simulink model "MRAC2016"  (R2016b)
settings: Solver=ode4  StartTime=0.0  StopTime=10  FixedStep=0.01  MaxStep=1e-3  RelTol=1e-3  AbsTol=1e-4
values from neighbouring files (symbols this model uses):
  A = [-3.1074 0.9744;0.4501 -4.1003]    [MRAC_params.m]
  A_hat_0 = [-5,0.2;0.1,-1]    [MRAC_params.m]
  Am = [-3.3808 1.2954;0.4444 -3.0501]    [MRAC_params.m]
  B = [B1,B2]    [MRAC_params.m]
  beta_1 = 100    [MRAC_params.m]
  Bm = [Bm1,Bm2]    [MRAC_params.m]
  d = [0.21;0.44]    [MRAC_params.m]
  d_hat_0 = [0.08;0.12]    [MRAC_params.m]
  dm = [0.1;0.3]    [MRAC_params.m]
  flag = 1    [MRAC_params.m]
  Gamma_A = 0.01*eye(2)    [MRAC_params.m]
  gamma_A = 0.0001    [MRAC_params.m]
  gamma_d = 1    [MRAC_params.m]
  P = are(Am,zeros(2,2),Q)    [MRAC_params.m]
  x_0 = [0.5;0.2]    [MRAC_params.m]
  xm_0 = [0;0]    [MRAC_params.m]
undefined symbols (not defined in the file or in its folder): sigbuilder_block
settings Model: Creator=RUZHOU  LastModifiedBy=Administrator
settings OptimizationCC: LifeSpan=inf
settings DebuggingCC: SFExecutionAtInitializationDiag=none
settings SFSimCC: SimUseLocalCustomCode=on
settings RTWCC: RTWUseLocalCustomCode=on

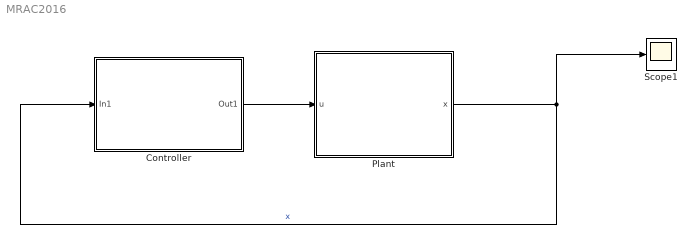
== system MRAC2016 ==
  Controller : Subsystem
  Plant : Subsystem
  Scope1 : Scope
  wires:
  Plant/1(x) -> Controller/1(In1), Scope1/1  "x"
  Controller/1(Out1) -> Plant/1(u)

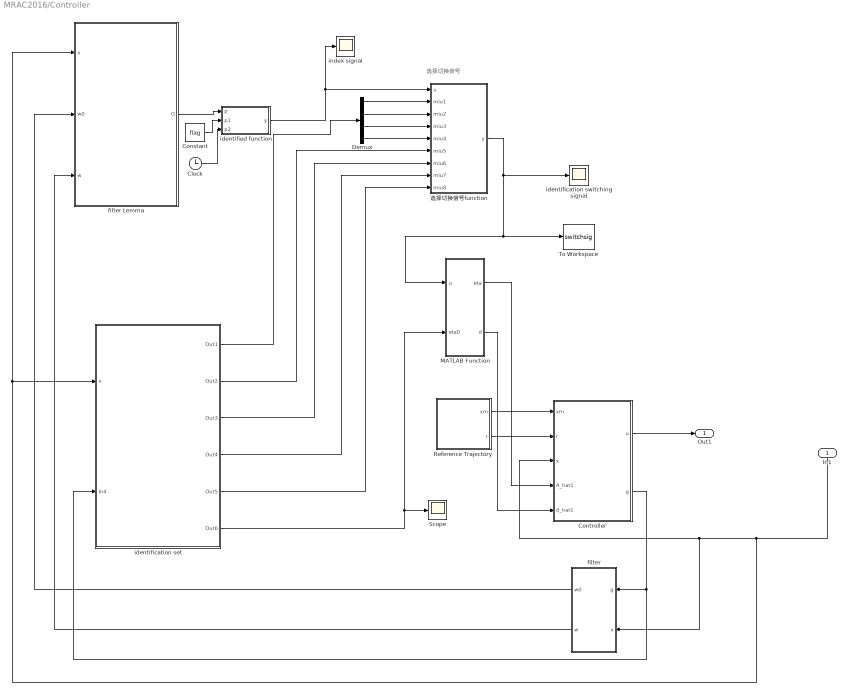
== system MRAC2016/Controller ==
  note: 选择切换信号
  In1 : Inport
  Clock : Clock
  Constant : Constant  Value=flag
  Controller : Subsystem
  Demux : Demux
  MATLAB Function : MATLAB Function  TreatAsAtomicUnit=on
  Reference Trajectory : Subsystem
  Scope : Scope
  To Workspace : ToWorkspace  VariableName=switchsig  SampleTime=-1
      settings: Save2DSignal=2-D array (concatenate along first dimension)
  filter : Subsystem
  filter Lemma : Subsystem
  identification set : Subsystem
  identification switching signal : Scope
  identified function : MATLAB Function  TreatAsAtomicUnit=on
  index signal : Scope
  选择切换信号function : MATLAB Function  TreatAsAtomicUnit=on
  Out1 : Outport
  wires:
  Demux/2 -> 选择切换信号function/3(miu2)
  Demux/3 -> 选择切换信号function/4(miu3)
  Reference Trajectory/2(r) -> Controller/2(r)
  Reference Trajectory/1(xm) -> Controller/1(xm)
  Controller/2(g) -> filter/1("g "), identification set/2(In4)
  Demux/1 -> 选择切换信号function/2(miu1)
  选择切换信号function/1(y) -> identification switching signal/1, To Workspace/1, MATLAB Function/1(u)
  identification set/5(Out5) -> 选择切换信号function/9(miu8)
  Constant/1 -> identified function/2(p1)
  Demux/4 -> 选择切换信号function/5(miu4)
  MATLAB Function/2(d) -> Controller/5(d_hat1)
  MATLAB Function/1(eta) -> Controller/4(A_hat1)
  identification set/1(Out1) -> Demux/1
  filter/1(w0) -> filter Lemma/2(w0)
  identified function/1(y) -> index signal/1, 选择切换信号function/1(u)
  filter/2(w) -> filter Lemma/3(w)
  filter Lemma/1(G) -> identified function/1(p)
  Clock/1 -> identified function/3(p2)
  identification set/4(Out4) -> 选择切换信号function/8(miu7)
  Controller/1(u) -> Out1/1
  identification set/6(Out6) -> Scope/1, MATLAB Function/2(eta0)
  identification set/2(Out2) -> 选择切换信号function/6(miu5)
  identification set/3(Out3) -> 选择切换信号function/7(miu6)
  In1/1 -> identification set/1(x), filter Lemma/1(x), Controller/3(x), filter/2(x)

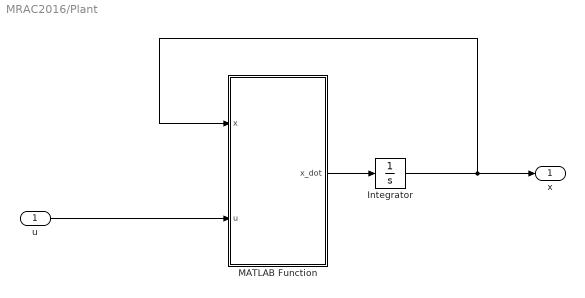
== system MRAC2016/Plant ==
  u : Inport
  Integrator : Integrator  InitialCondition=x_0  LimitOutput=on  UpperSaturationLimit=1000  LowerSaturationLimit=-1000
  MATLAB Function : MATLAB Function  TreatAsAtomicUnit=on
  x : Outport
  wires:
  MATLAB Function/1(x_dot) -> Integrator/1
  Integrator/1 -> MATLAB Function/1(x), x/1
  u/1 -> MATLAB Function/2(u)

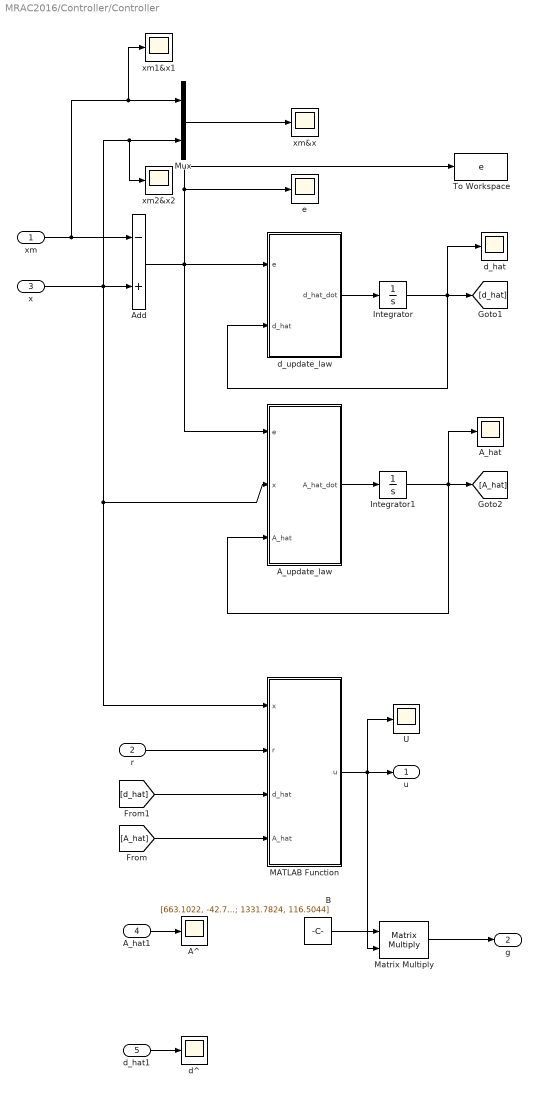
== system MRAC2016/Controller/Controller ==
  xm : Inport
  r : Inport  Port=2
  x : Inport  Port=3
  A_hat1 : Inport  Port=4
  d_hat1 : Inport  Port=5
  A^ : Scope
  A_hat : Scope
  A_update_law : MATLAB Function  TreatAsAtomicUnit=on
  Add : Sum  Inputs=-+
  B : Constant  Value=[663.1022, -42.7; 1331.7824, 116.5044]  VectorParams1D=off
  Integrator : Integrator  InitialCondition=d_hat_0
  Integrator1 : Integrator  InitialCondition=A_hat_0
  MATLAB Function : MATLAB Function  TreatAsAtomicUnit=on
  Matrix Multiply : Product  Multiplication=Matrix(*)
  Mux : Mux  Inputs=2
  To Workspace : ToWorkspace  VariableName=e  SaveFormat=Timeseries  SampleTime=-1
  U : Scope
  d^ : Scope
  d_hat : Scope
  d_update_law : MATLAB Function  TreatAsAtomicUnit=on
  e : Scope
  xm&x : Scope
  xm1&x1 : Scope
  xm2&x2 : Scope
  u : Outport
  g : Outport  Port=2
  wires:
  x/1 -> xm2&x2/1, Mux/2, MATLAB Function/1(x), A_update_law/2(x), Add/2
  xm/1 -> xm1&x1/1, Mux/1, Add/1
  Add/1 -> To Workspace/1, e/1, A_update_law/1(e), d_update_law/1(e)
  d_update_law/1(d_hat_dot) -> Integrator/1
  Integrator/1 -> d_hat/1, d_update_law/2(d_hat), [d_hat]
  A_update_law/1(A_hat_dot) -> Integrator1/1
  Integrator1/1 -> A_update_law/3(A_hat), [A_hat], A_hat/1
  r/1 -> MATLAB Function/2(r)
  [d_hat] -> MATLAB Function/3(d_hat)
  MATLAB Function/1(u) -> Matrix Multiply/2, U/1, u/1
  Mux/1 -> xm&x/1
  B/1 -> Matrix Multiply/1
  Matrix Multiply/1 -> g/1
  A_hat1/1 -> A^/1
  d_hat1/1 -> d^/1
  [A_hat] -> MATLAB Function/4(A_hat)

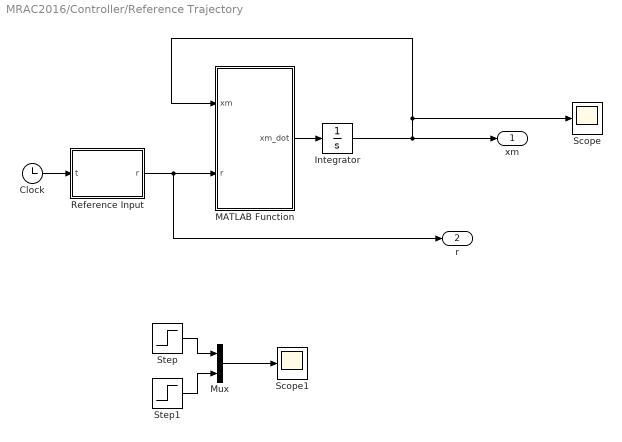
== system MRAC2016/Controller/Reference Trajectory ==
  Clock : Clock
  Integrator : Integrator  InitialCondition=xm_0
  MATLAB Function : MATLAB Function  TreatAsAtomicUnit=on
  Mux : Mux  Inputs=2
  Reference Input : MATLAB Function  TreatAsAtomicUnit=on
  Scope : Scope
  Scope1 : Scope
  Step : Step  SampleTime=0
  Step1 : Step  SampleTime=0
  xm : Outport
  r : Outport  Port=2
  wires:
  MATLAB Function/1(xm_dot) -> Integrator/1
  Clock/1 -> Reference Input/1(t)
  Integrator/1 -> Scope/1, MATLAB Function/1(xm), xm/1
  Reference Input/1(r) -> r/1, MATLAB Function/2(r)
  Step/1 -> Mux/1
  Step1/1 -> Mux/2
  Mux/1 -> Scope1/1

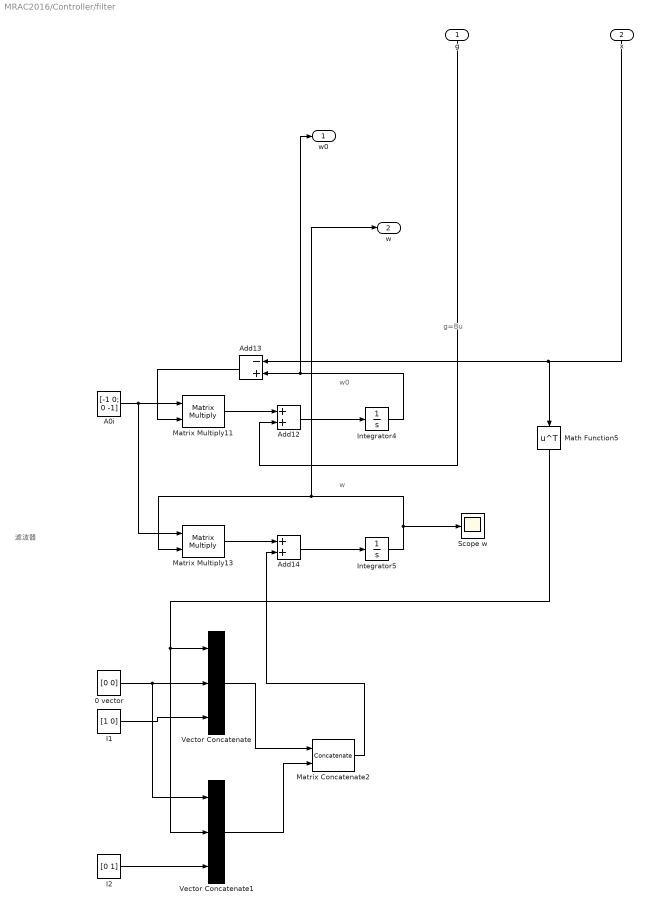
== system MRAC2016/Controller/filter ==
  note: w0
  note: 滤波器
  note: g=Bu
  note: w
  "g " : Inport
  x : Inport  Port=2
  0 vector : Constant  Value=[0 0]  VectorParams1D=off
  A0i : Constant  Value=[-1 0; 0 -1]  VectorParams1D=off
  Add12 : Sum
  Add13 : Sum  Inputs=-+
  Add14 : Sum
  I1 : Constant  Value=[1 0]  VectorParams1D=off
  I2 : Constant  Value=[0 1]  VectorParams1D=off
  Integrator4 : Integrator
  Integrator5 : Integrator
  Math Function5 : Math  Operator=transpose  SaturateOnIntegerOverflow=on
  Matrix Concatenate2 : Concatenate  Mode=Multidimensional array
  Matrix Multiply11 : Product  Multiplication=Matrix(*)
  Matrix Multiply13 : Product  Multiplication=Matrix(*)
  Scope w : Scope
  Vector Concatenate : Concatenate  NumInputs=3
  Vector Concatenate1 : Concatenate  NumInputs=3
  w0 : Outport
  w : Outport  Port=2
  wires:
  Math Function5/1 -> Vector Concatenate1/2, Vector Concatenate/1
  Matrix Multiply11/1 -> Add12/1
  I2/1 -> Vector Concatenate1/3
  Vector Concatenate/1 -> Matrix Concatenate2/1
  I1/1 -> Vector Concatenate/3
  Add12/1 -> Integrator4/1
  Matrix Multiply13/1 -> Add14/1
  Integrator4/1 -> w0/1, Add13/2
  Integrator5/1 -> w/1, Matrix Multiply13/2, Scope w/1
  Matrix Concatenate2/1 -> Add14/2
  0 vector/1 -> Vector Concatenate1/1, Vector Concatenate/2
  Vector Concatenate1/1 -> Matrix Concatenate2/2
  Add13/1 -> Matrix Multiply11/2
  Add14/1 -> Integrator5/1
  A0i/1 -> Matrix Multiply13/1, Matrix Multiply11/1
  x/1 -> Math Function5/1, Add13/1
  "g "/1 -> Add12/2

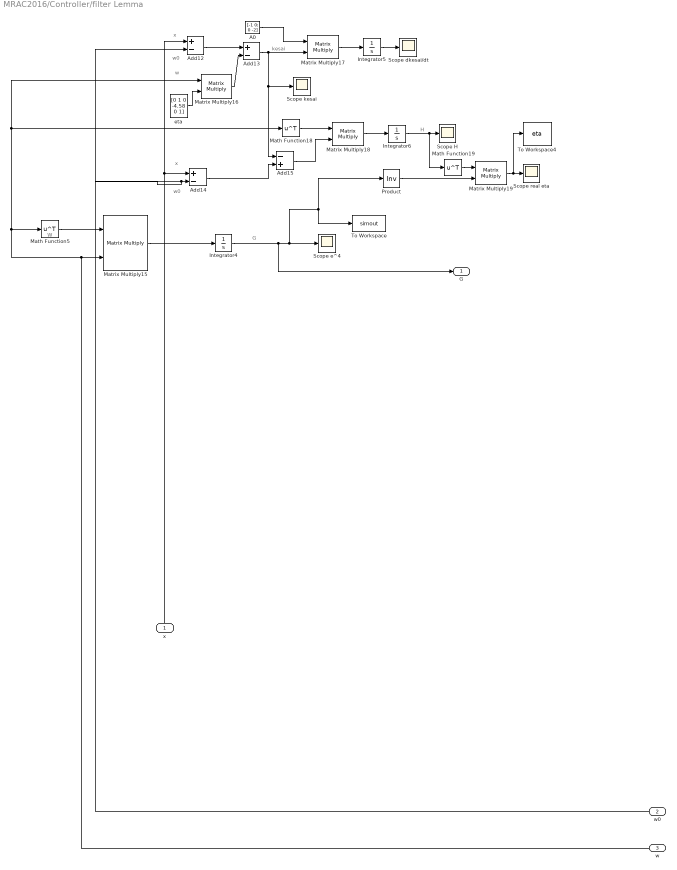
== system MRAC2016/Controller/filter Lemma ==
  note: H
  note: w0
  note: x
  note: kesai
  note: w
  note: w0
  note: x
  note: W
  note: G
  x : Inport
  w0 : Inport  Port=2
  w : Inport  Port=3
  A0 : Constant  Value=[-1 0; 0 -2]
  Add12 : Sum  Inputs=+-
  Add13 : Sum  Inputs=+-
  Add14 : Sum  Inputs=+-
  Add15 : Sum  Inputs=-+
  Integrator4 : Integrator
  Integrator5 : Integrator
  Integrator6 : Integrator
  Math Function18 : Math  Operator=transpose  SaturateOnIntegerOverflow=on
  Math Function19 : Math  Operator=transpose  SaturateOnIntegerOverflow=on
  Math Function5 : Math  Operator=transpose  SaturateOnIntegerOverflow=on
  Matrix Multiply{15..19} (5 alike) : Product  Multiplication=Matrix(*)
  Product : Product  Inputs=/  Multiplication=Matrix(*)
  Scope H : Scope
  Scope dkesai/dt : Scope
  Scope e^4 : Scope
  Scope kesai : Scope
  Scope real eta : Scope
  To Workspace : ToWorkspace  VariableName=simout  SaveFormat=Timeseries  SampleTime=-1
  To Workspace4 : ToWorkspace  VariableName=eta  SampleTime=-1
      settings: Save2DSignal=2-D array (concatenate along first dimension)
  eta : Constant  Value=[0 1 0 -4.58 0 1]
  G : Outport
  wires:
  w0/1 -> Add12/2, Add14/2
  w/1 -> Math Function18/1, Matrix Multiply16/1, Math Function5/1, Matrix Multiply15/2
  eta/1 -> Matrix Multiply16/2
  Add15/1 -> Matrix Multiply18/2
  Matrix Multiply15/1 -> Integrator4/1
  Matrix Multiply17/1 -> Integrator5/1
  Add12/1 -> Add13/1
  Integrator5/1 -> Scope dkesai/dt/1
  Product/1 -> Matrix Multiply19/2
  Integrator4/1 -> G/1, Product/1, To Workspace/1, Scope e^4/1
  Math Function5/1 -> Matrix Multiply15/1
  Add13/1 -> Scope kesai/1, Add15/1, Matrix Multiply17/2
  Add14/1 -> Add15/2
  Math Function18/1 -> Matrix Multiply18/1
  Matrix Multiply18/1 -> Integrator6/1
  Integrator6/1 -> Math Function19/1, Scope H/1
  Math Function19/1 -> Matrix Multiply19/1
  Matrix Multiply16/1 -> Add13/2
  A0/1 -> Matrix Multiply17/1
  Matrix Multiply19/1 -> To Workspace4/1, Scope real eta/1
  x/1 -> Add12/1, Add14/1

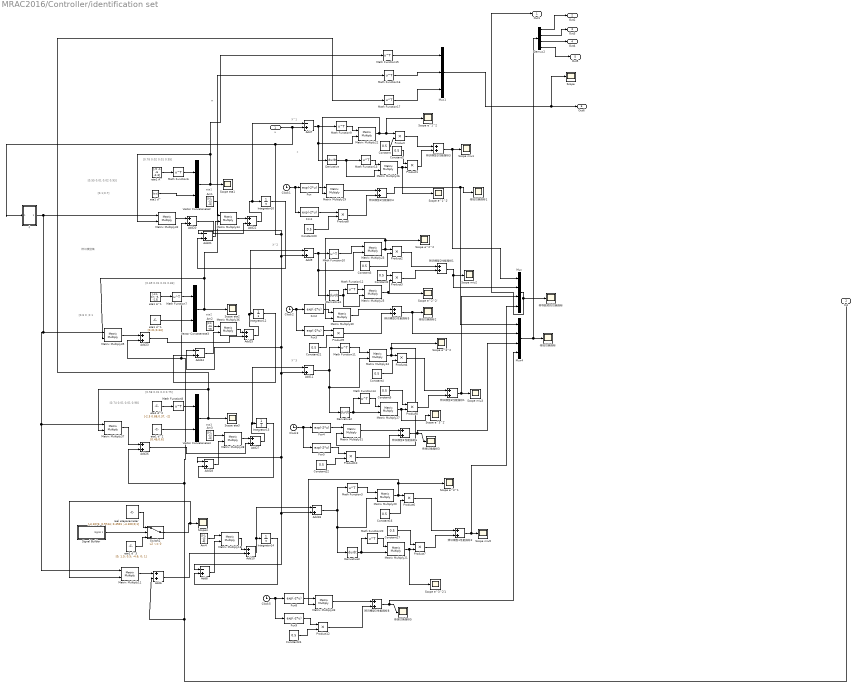
== system MRAC2016/Controller/identification set ==
  note: [0.58 0.01 0.0 0.75]
  note: [0.69 0.01 0.01 0.83]
  note: [0.78 0.02 0.01 0.95]
  note: x
  note: [0.8 0 ;0 1
  note: [0.1;0.7]
  note: [0.55 0.01 0.02 0.93]
  note: [0.74 0.01 0.01 0.98]
  note: w
  note: 辨识模型集
  note: X^3
  note: X^2
  note: X^1
  note: eta1
  note: eta2
  note: eta3
  x : Inport
  In4 : Inport  Port=2
  " 带导数项的切换指标" : Scope
  Add{6,10,20,22..23,25..27} (8 alike) : Sum
  Add{7..9,11,18,21,24,28} (8 alike) : Sum  Inputs=-+
  Am{1..4} (4 alike) : Constant  Value=[0 1; -15 -8]  VectorParams1D=off
  Clock{1..3,5} (4 alike) : Clock
      settings: Decimation=50
  Constant{,1..5,16..17,20..22,24} (12 alike) : Constant  Value=0.5
  Demux2 : Demux
  Derivative{,1..3} (4 alike) : Derivative
  Fcn{,1..5,8..9} (8 alike) : Fcn  Expr=exp(-2*u)
  Integrator{10,12..14} (4 alike) : Integrator
  Math Function{3,6..17,20} (14 alike) : Math  Operator=transpose  SaturateOnIntegerOverflow=on
  Matrix Multiply{11,13,20..27,29..38} (20 alike) : Product  Multiplication=Matrix(*)
  Mux : Mux
  Mux1 : Mux  Inputs=3
  Mux4 : Mux
  Product{,1..10,12} (12 alike) : Product
  Scope : Scope
  Scope e^1^2 : Scope
  Scope e^1^2' : Scope
  Scope e^2^2 : Scope
  Scope e^2^2' : Scope
  Scope e^3^1 : Scope
  Scope e^3^2 : Scope
  Scope e^3^2' : Scope
  Scope e^3^2'1 : Scope
  Scope eta1 : Scope
  Scope eta2 : Scope
  Scope eta3 : Scope
  Scope miu{1..3,5} (4 alike) : Scope
  Scope4 : Scope
  Signal Builder : Subsystem  Tag=STV Subsys  LoadFcn=sigbuilder_block('load');  StartFcn=sigbuilder_block('start');  StopFcn=sigbuilder_block('stop');  ClipboardFcn=sigbuilder_block('clipboard');  mask(Sigbuilder block){tuvar=[0:10]}
      mask help: Simulink:masks:SigbuilderBlock_MD
      mask init:
      | if ~strcmp(get_param(bdroot(gcbh),'SimulationStatus'),'stopped') tuvar = sigbuilder_block('maskInit'); end
      settings: CopyFcn=sigbuilder_block('copy');  DeleteFcn=sigbuilder_block('delete');  ModelCloseFcn=sigbuilder_block('modelClose');  PreSaveFcn=sigbuilder_block('preSave');  PauseFcn=sigbuilder_block('pause');  ContinueFcn=sigbuilder_block('continue');  NameChangeFcn=sigbuilder_block('namechange');  OpenFcn=sigbuilder_block('open',[646.5 180.75 550.5 399.75 ]);  CloseFcn=sigbuilder_block('close');
      mask Display: plot(0, 0, 100, 100,[2, 2, 32, 32, 2], [68, 8, 8, 68, 68],[32, 2], [38, 38], [32, 19, 2],[53, 60, 44], [32, 17, 17, 2],[16, 16, 31, 31]);txt = getActiveGroup(gcbh);text(2, 100, txt,'verticalAlignment', 'top');
  Switch2 : Switch  Criteria=u2 ~= 0
  Vector Concatenate2 : Concatenate
  Vector Concatenate3 : Concatenate
  Vector Concatenate4 : Concatenate
  eta1 A^ : Constant  Value=[-5 -1 -6 -2.3]  VectorParams1D=off
  eta1 A^1 : Constant  Value=[-2.1, 0.7, -5, -2.3]  VectorParams1D=off
  eta1 A^2 : Constant  Value=[-2.5 0.88,0.37, -2]  VectorParams1D=off
  eta1 d^ : Constant  Value=[0;0]  VectorParams1D=off
  eta1 d^1 : Constant  Value=[0.21;0.34]  VectorParams1D=off
  eta1 d^2 : Constant  Value=[0.45;0.6]  VectorParams1D=off
  eta1 d^3 : Constant  Value=[0; 1.5; 0.5; -4.6; 0; 1]  VectorParams1D=off
  f : Subsystem
  "real etaparameter " : Constant  Value=[-3.1074; 0.9744; 0.4501 ;-4.100;0;1]
  传统切换指标{,1..3,5} (5 alike) : Scope
  辨识模型2性能指标1 : Sum
  辨识模型3性能指标{1..6,8} (7 alike) : Sum
  Out1 : Outport
  Out2 : Outport  Port=2
  Out3 : Outport  Port=3
  Out4 : Outport  Port=4
  Out5 : Outport  Port=5
  Out6 : Outport  Port=6
  wires:
  x/1 -> Add21/1, Add24/1, Add28/1, Add8/1, Add18/2, Add11/2, Add9/2, f/1(In1), Add7/2
  eta1 d^1/1 -> Vector Concatenate3/2
  eta1 A^2/1 -> Math Function8/1
  Math Function8/1 -> Vector Concatenate4/1
  eta1 d^2/1 -> Vector Concatenate4/2
  Math Function6/1 -> Vector Concatenate2/1
  eta1 A^/1 -> Math Function6/1
  eta1 A^1/1 -> Math Function7/1
  Math Function7/1 -> Vector Concatenate3/1
  eta1 d^/1 -> Vector Concatenate2/2
  Vector Concatenate3/1 -> Scope eta2/1, Matrix Multiply35/2, Math Function16/1
  Add7/1 -> Math Function9/1, Matrix Multiply22/2, Derivative/1
  Math Function9/1 -> Matrix Multiply22/1
  Add9/1 -> Matrix Multiply23/2, Derivative1/1, Math Function10/1
  Math Function10/1 -> Matrix Multiply23/1
  Add11/1 -> Derivative2/1, Matrix Multiply24/2, Math Function11/1
  Math Function11/1 -> Matrix Multiply24/1
  Derivative1/1 -> Math Function12/1, Matrix Multiply25/2
  Math Function12/1 -> Matrix Multiply25/1
  Math Function13/1 -> Matrix Multiply26/1
  Math Function14/1 -> Matrix Multiply27/1
  Derivative/1 -> Matrix Multiply26/2, Math Function13/1
  Derivative2/1 -> Math Function14/1, Matrix Multiply27/2
  辨识模型3性能指标1/1 -> Mux/3, Scope miu3/1
  辨识模型3性能指标3/1 -> Mux/1, Scope miu1/1
  Mux/1 -> Out1/1, " 带导数项的切换指标"/1
  辨识模型2性能指标1/1 -> Mux/2, Scope miu2/1
  Vector Concatenate2/1 -> Matrix Multiply32/2, Math Function15/1, Scope eta1/1
  Vector Concatenate4/1 -> Matrix Multiply37/2, Math Function17/1, Scope eta3/1
  Mux1/1 -> Scope/1, Out6/1
  Math Function16/1 -> Mux1/2
  Math Function15/1 -> Mux1/1
  Math Function17/1 -> Mux1/3
  Matrix Multiply22/1 -> Matrix Multiply29/2, Scope e^1^2/1, Product/1
  Product/1 -> 辨识模型3性能指标3/1
  Constant/1 -> Product/2
  Matrix Multiply26/1 -> Scope e^1^2'/1, Product1/2
  Matrix Multiply23/1 -> Matrix Multiply30/2, Scope e^2^2/1, Product2/1
  Product1/1 -> 辨识模型3性能指标3/2
  Constant1/1 -> Product1/1
  Product2/1 -> 辨识模型2性能指标1/1
  Constant2/1 -> Product3/1
  Matrix Multiply25/1 -> Scope e^2^2'/1, Product3/2
  Constant4/1 -> Product4/2
  Matrix Multiply27/1 -> Scope e^3^2'/1, Product5/2
  Constant5/1 -> Product5/1
  Product3/1 -> 辨识模型2性能指标1/2
  Product4/1 -> 辨识模型3性能指标1/1
  Product5/1 -> 辨识模型3性能指标1/2
  Matrix Multiply24/1 -> Matrix Multiply31/2, Scope e^3^2/1, Product4/1
  Constant3/1 -> Product2/2
  Derivative3/1 -> Matrix Multiply21/2, Math Function20/1
  Matrix Multiply21/1 -> Product7/2, Scope e^3^2'1/1
  Add18/1 -> Math Function3/1, Matrix Multiply20/2, Derivative3/1
  Math Function3/1 -> Matrix Multiply20/1
  Constant17/1 -> Product7/1
  Product7/1 -> 辨识模型3性能指标2/2
  Product6/1 -> 辨识模型3性能指标2/1
  辨识模型3性能指标2/1 -> Mux/4, Scope miu5/1
  Math Function20/1 -> Matrix Multiply21/1
  Constant16/1 -> Product6/2
  Constant20/1 -> Product8/2
  辨识模型3性能指标4/1 -> Mux4/1, 传统切换指标1/1
  Clock2/1 -> Fcn3/1, Fcn2/1
  Fcn3/1 -> Product9/1
  Product8/1 -> 辨识模型3性能指标4/2
  Fcn1/1 -> Product8/1
  Clock1/1 -> Fcn1/1, Fcn/1
  Fcn2/1 -> Matrix Multiply30/1
  Matrix Multiply29/1 -> 辨识模型3性能指标4/1
  Fcn/1 -> Matrix Multiply29/1
  Constant21/1 -> Product9/2
  Matrix Multiply30/1 -> 辨识模型3性能指标5/1
  Product9/1 -> 辨识模型3性能指标5/2
  Fcn5/1 -> Product10/1
  Product10/1 -> 辨识模型3性能指标6/2
  Matrix Multiply31/1 -> 辨识模型3性能指标6/1
  辨识模型3性能指标5/1 -> Mux4/2, 传统切换指标2/1
  Fcn8/1 -> Matrix Multiply33/1
  辨识模型3性能指标6/1 -> Mux4/3, 传统切换指标3/1
  Clock5/1 -> Fcn9/1, Fcn8/1
  Constant22/1 -> Product10/2
  Matrix Multiply20/1 -> Product6/1, Matrix Multiply33/2, Scope e^3^1/1
  Fcn9/1 -> Product12/1
  Clock3/1 -> Fcn5/1, Fcn4/1
  Fcn4/1 -> Matrix Multiply31/1
  f/1(Out1) -> Matrix Multiply11/1, Matrix Multiply37/1, Matrix Multiply35/1, Matrix Multiply32/1
  Demux2/3 -> Out4/1
  Matrix Multiply32/1 -> Add20/1
  Switch2/1 -> Matrix Multiply11/2, Scope4/1
  Am1/1 -> Matrix Multiply34/1
  Integrator10/1 -> Add21/2
  Product12/1 -> 辨识模型3性能指标8/2
  辨识模型3性能指标8/1 -> Mux4/4, 传统切换指标5/1
  "real etaparameter "/1 -> Switch2/1
  Mux4/1 -> Demux2/1, 传统切换指标/1
  Demux2/1 -> Out2/1
  Demux2/4 -> Out5/1
  eta1 d^3/1 -> Switch2/3
  Constant24/1 -> Product12/2
  Matrix Multiply33/1 -> 辨识模型3性能指标8/1
  Demux2/2 -> Out3/1
  Signal Builder/1(Signal 1) -> Switch2/2
  Matrix Multiply34/1 -> Add22/1
  Add20/1 -> Add22/2
  Am2/1 -> Matrix Multiply36/1
  Add21/1 -> Matrix Multiply34/2
  Integrator12/1 -> Add24/2
  Matrix Multiply36/1 -> Add25/1
  Add25/1 -> Add9/1, Integrator12/1
  Matrix Multiply35/1 -> Add23/1
  Add22/1 -> Add7/1, Integrator10/1
  Add24/1 -> Matrix Multiply36/2
  In4/1 -> Add6/2, Add26/2, Add23/2, Add20/2
  Add10/1 -> Add18/1, Integrator14/1
  Am3/1 -> Matrix Multiply38/1
  Add28/1 -> Matrix Multiply38/2
  Integrator13/1 -> Add28/2
  Integrator14/1 -> Add8/2
  Add23/1 -> Add25/2
  Matrix Multiply37/1 -> Add26/1
  Add27/1 -> Add11/1, Integrator13/1
  Matrix Multiply11/1 -> Add6/1
  Am4/1 -> Matrix Multiply13/1
  Matrix Multiply38/1 -> Add27/1
  Add8/1 -> Matrix Multiply13/2
  Add26/1 -> Add27/2
  Add6/1 -> Add10/2
  Matrix Multiply13/1 -> Add10/1

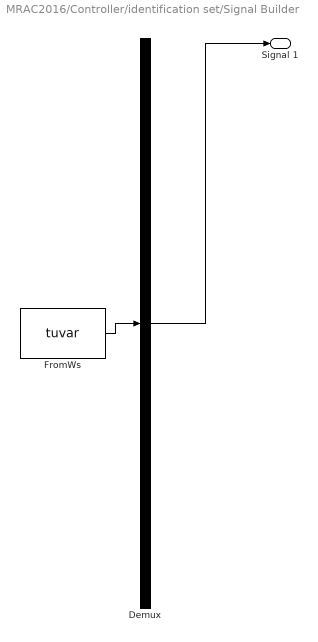
== system MRAC2016/Controller/identification set/Signal Builder ==
  Demux : Demux  Tag=STV Demux  Outputs=1
  FromWs : FromWorkspace  Tag=STV FromWs  VariableName=tuvar  SampleTime=0
      SigBuilderData=|
      | common.afterFinalStr = 'Extrapolate'
      | common.sampleTime = 0
      | dataSet.timeRange = [0 10]
      | dataSet.name = 'Group 1'
      | sbobj.Groups.Name = 'Group 1'
      | sbobj.Groups.Signals.Name = 'Signal 1'
      | sbobj.Groups.Signals.XData = [0 6 10]
      | sbobj.Groups.Signals.YData = [1 1 1]
  Signal 1 : Outport  Tag=STV Outport
  wires:
  Demux/1 -> Signal 1/1
  FromWs/1 -> Demux/1

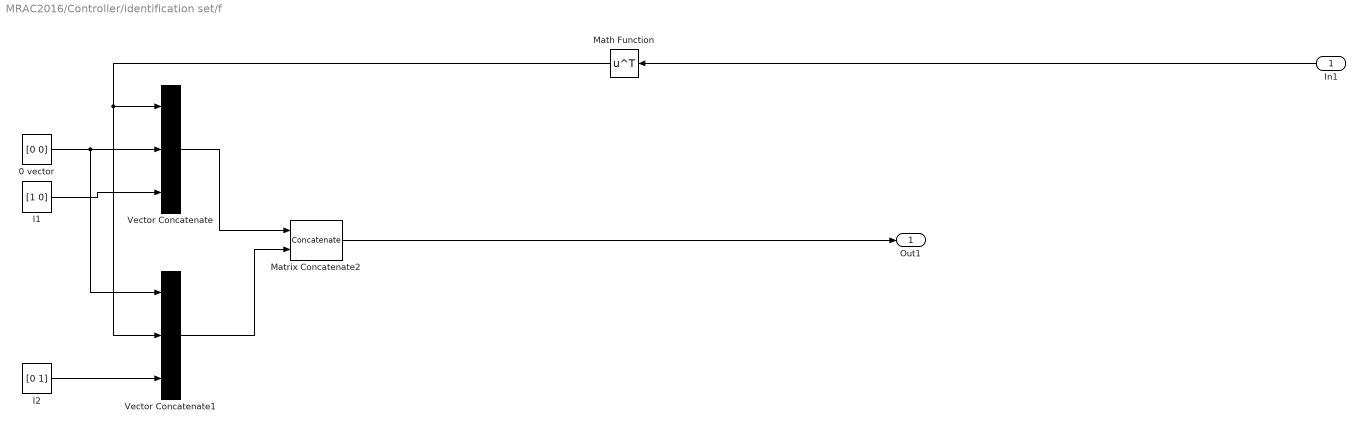
== system MRAC2016/Controller/identification set/f ==
  In1 : Inport
  0 vector : Constant  Value=[0 0]  VectorParams1D=off
  I1 : Constant  Value=[1 0]  VectorParams1D=off
  I2 : Constant  Value=[0 1]  VectorParams1D=off
  Math Function : Math  Operator=transpose  SaturateOnIntegerOverflow=on
  Matrix Concatenate2 : Concatenate  Mode=Multidimensional array
  Vector Concatenate : Concatenate  NumInputs=3
  Vector Concatenate1 : Concatenate  NumInputs=3
  Out1 : Outport
  wires:
  In1/1 -> Math Function/1
  0 vector/1 -> Vector Concatenate1/1, Vector Concatenate/2
  I1/1 -> Vector Concatenate/3
  Vector Concatenate1/1 -> Matrix Concatenate2/2
  I2/1 -> Vector Concatenate1/3
  Vector Concatenate/1 -> Matrix Concatenate2/1
  Matrix Concatenate2/1 -> Out1/1
  Math Function/1 -> Vector Concatenate1/2, Vector Concatenate/1

== matlab function MRAC2016/Controller/Controller/d_update_law ==
  data: e input; d_hat_dot output; d_hat input; beta_1 parameter; P parameter; gamma_d parameter
function d_hat_dot = fcn(e,d_hat,beta_1, P, gamma_d)

d_hat_dot = beta_1*P*e - gamma_d*d_hat;
end

== matlab function MRAC2016/Plant/MATLAB Function ==
  data: x input; u input; x_dot output; A parameter; B parameter; d parameter
function x_dot = fcn(x,u,A, B, d)

x_dot = A*x + B*u + d;
end

== matlab function MRAC2016/Controller/Controller/A_update_law ==
  data: e input; A_hat_dot output; x input; Gamma_A parameter; P parameter; A_hat input; gamma_A parameter
function A_hat_dot = fcn(e,x,Gamma_A, P, A_hat, gamma_A)
A_hat_dot = Gamma_A*P*e*x' - gamma_A*A_hat;
end

== matlab function MRAC2016/Controller/Controller/MATLAB Function ==
  data: x input; u output; r input; d_hat input; A_hat input; Bm parameter; dm parameter; Am parameter; B parameter
function u = fcn(x,r,d_hat,A_hat,Bm, dm, Am, B)

u = B\(Bm*r - (d_hat - dm) - (A_hat - Am)*x);
end

== matlab function MRAC2016/Controller/Reference Trajectory/MATLAB Function ==
  data: xm input; xm_dot output; r input; Am parameter; Bm parameter; dm parameter
function xm_dot = fcn(xm,r,Am, Bm, dm)

xm_dot = Am*xm + Bm*r + dm;
end

== matlab function MRAC2016/Controller/Reference Trajectory/Reference Input ==
  data: t input; r output
function r = fcn(t)

r = [0.1*sin(0.1*2*pi*t)+0.15;
    0.06*sin(0.2*2*pi*t)+0.1];
end

== matlab function MRAC2016/Controller/MATLAB Function ==
  data: u input; eta output; eta0 input; d output
function [eta,d] = fcn(u,eta0)
    if u == -1
        eta = [0,0;0,0];
        d = [0;0];
    elseif u == 1
        eta = [eta0(1),eta0(2);eta0(3),eta0(4)];
        d = [eta0(5);eta0(6)];
    elseif u == 2
        eta = [eta0(7),eta0(8);eta0(9),eta0(10)];
        d = [eta0(11);eta0(12)];
    elseif u == 3
        eta = [eta0(13),eta0(14);eta0(15),eta0(16)];
        d = [eta0(17);eta0(18)];
    else
        eta = [0,0;0,0];
        d = [0;0];
    end

== matlab function MRAC2016/Controller/选择切换信号function ==
  data: u input; y output; miu1 input; miu2 input; miu3 input; miu4 input; miu5 input; miu6 input; miu7 input; miu8 input
function y = fcn(u,miu1,miu2,miu3,miu4,miu5,miu6,miu7,miu8)
    if (u == 1)
        n = [miu1, miu2, miu3, miu4];
        miu = min(n);
        if (miu == miu1)
            miu = 1;
        end
        if(miu == miu2)
            miu = 2;
        end
        if(miu == miu3)
            miu = 3;
        end
        if(miu == miu4)
            miu = 4;
        end
    else
        n = [miu5, miu6, miu7, miu8];
        miu = min(n);
        if (miu == miu5)
            miu = 1;
        end
        if (miu == miu6)
            miu = 2;
        end
        if (miu == miu7)
            miu = 3;
        end
        if(miu == miu8)
            miu = 4;
        end
    end
y = miu;

== matlab function MRAC2016/Controller/identified function ==
  data: p input; y output; p1 input; p2 input
function y = fcn(p,p1,p2)
    if (p1 == 0 && p2 < 0)
        u = 2;
    else
        u = 1;
    end
y = u;
